simulink model "pidtrack_demo"  (Simulink 6.0)
settings: Solver=ode45  StartTime=0.0  StopTime=100  RelTol=1e-3  AbsTol=1e-6
PreLoadFcn:
  | load pidtrack_demo
undefined symbols (not defined in the file or in its folder): a1, a2, Kd, Ki, Kp
libraries: srolib x1
settings Model: Creator=ksubbara  LastModifiedBy=pascal  ModelDataFile=srodemo1.mat
settings DataIOCC: SignalLoggingName=DataLog
settings DebuggingCC: CheckExecutionContextPreStartOutputMsg=on  CheckExecutionContextRuntimeOutputMsg=on  SolverPrmCheckMsg=none
settings HardwareCC: TargetUnknown=on
settings ModelReferenceCC: UpdateModelReferenceTargets=IfOutOfDate
settings GRTTargetCC: LifeSpan=inf
settings SFSimCC: SFSimApplyToAllLibs=on  SFSimBuildMode=Incremental

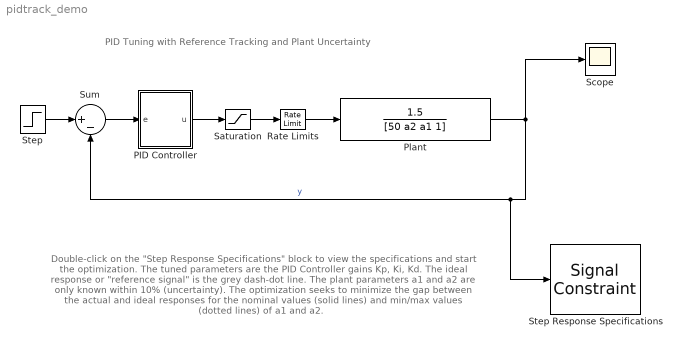
== system pidtrack_demo ==
  note: PID Tuning with Reference Tracking and Plant Uncertainty
  note: Double-click on the "Step Response Specifications" block to view the
      | specifications and start the optimization.
      |
      | The tuned parameters are the PID Controller gains Kp, Ki, Kd.
      | The ideal response or "reference signal" is the grey dash-dot line.
      | The plant parameters a1 and a2 are only known within 10% (uncertainty).
      |
      | The optimization seeks to minimize the gap between the actual and ideal responses
      | for the nominal values (solid lines) and min/max values (dotted lines) of a1 and a2.
  PID Controller : Subsystem  PropExecContextAcrossSSBoundary=on
  Plant : TransferFcn  Numerator=[1.5]  Denominator=[50 a2 a1 1]
  Rate Limits : RateLimiter  RisingSlewLimit=0.8  FallingSlewLimit=-0.8
  Saturation : Saturate  UpperLimit=2  LowerLimit=-2
  Scope : Scope
  Step : Step  Time=0  SampleTime=0
  Step Response Specifications : srolib/Signal Constraint  DialogPosition=[0.016875 0.36 0.37875 0.270833333333333]  SaveIn=workspace  SaveAs=pidtrack_optim  LogID=SRO_DataLog_1
  Sum : Sum  Inputs=|+-  SaturateOnIntegerOverflow=on
  wires:
  Sum/1 -> PID Controller/1(e)
  Step/1 -> Sum/1
  Saturation/1 -> Rate Limits/1
  Rate Limits/1 -> Plant/1
  PID Controller/1(u) -> Saturation/1
  Plant/1 -> Scope/1, Sum/2, Step Response Specifications/1  "y"

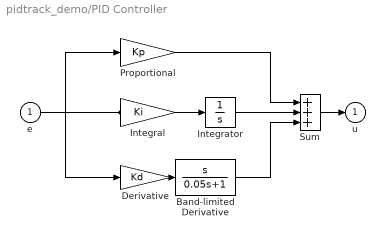
== system pidtrack_demo/PID Controller ==
  e : Inport  LatchInput=off
  Band-limited Derivative : TransferFcn  Numerator=[1 0]  Denominator=[0.05 1]
  Derivative : Gain  Gain=Kd  SaturateOnIntegerOverflow=on
  Integral : Gain  Gain=Ki  SaturateOnIntegerOverflow=on
  Integrator : Integrator
  Proportional : Gain  Gain=Kp  SaturateOnIntegerOverflow=on
  Sum : Sum  Inputs=+++  SaturateOnIntegerOverflow=on  InputSameDT=on
  u : Outport  InitialOutput=0
  wires:
  Integrator/1 -> Sum/2
  Derivative/1 -> Band-limited Derivative/1
  Sum/1 -> u/1
  e/1 -> Integral/1, Proportional/1, Derivative/1
  Band-limited Derivative/1 -> Sum/3
  Integral/1 -> Integrator/1
  Proportional/1 -> Sum/1
